simulink model "controls"  (R2022b)
settings: Solver=FixedStepAuto  StartTime=0.0  StopTime=inf  FixedStep=0.001  RelTol=1e-3
libraries: canmsglib x11, speedgoatlib_IO614 x5, speedgoatlib_CAN x1, battery_monitor_lib x1, driver_interface_lib x1, governor_lib x1, motor_interface_lib x1, simp_vd_lib x1
settings Model: Creator=maxfa  LastModifiedBy=maxfa
settings SolverCC: ConcurrentTasks=on  PositivePriorityOrder=on
settings OptimizationCC: BlockReduction=off  OptimizeBlockIOStorage=off
settings DebuggingCC: TasksWithSamePriorityMsg=none
settings HardwareCC: ProdBitPerLong=64  ProdLongLongMode=on  ProdHWDeviceType=Intel->x86-64 (Linux 64)
settings RTWCC: Description=Simulink Real-Time  SystemTargetFile=slrealtime.tlc  TemplateMakefile=slrealtime_default_tmf  Toolchain=Simulink Real-Time Toolchain  BuildConfiguration=Faster Runs  CodeExecutionProfiling=on  TargetLang=C++

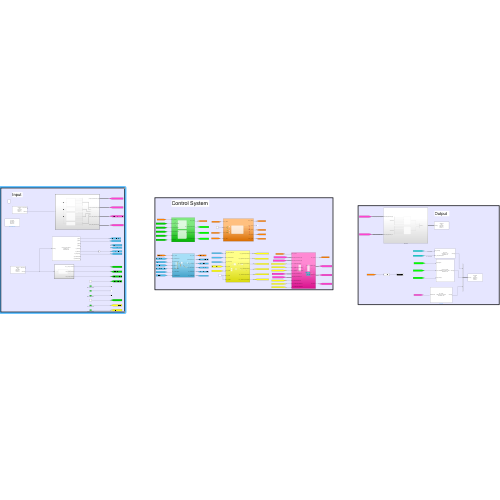
[thumbnail: Simulink's stored preview of the top-level diagram]
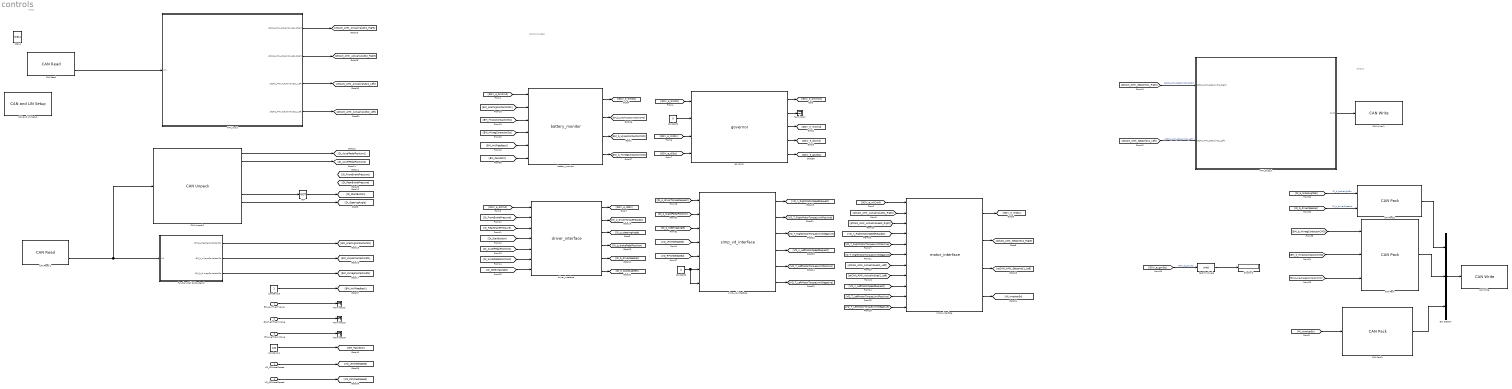
== system controls ==
  note: Control System
  note: Input
  note: Output
  BM_LowThermValue : Inport  OutDataTypeStr=int8  Unit=°C
  BM_HighThermValue : Inport  Port=2  OutDataTypeStr=int8  Unit=°C
  BM_AvgThermValue : Inport  Port=3  OutDataTypeStr=int8  Unit=°C
  VD_LFWheelSpeed : Inport  Port=4  OutDataTypeStr=int16  Unit=rpm
  VD_RFWheelSpeed : Inport  Port=5  OutDataTypeStr=int16  Unit=rpm
  AMK_Input : Subsystem  TreatAsAtomicUnit=on
  AMK_Output : Subsystem
  Bus Creator : BusCreator  Inputs=3
  CAN Pack : canmsglib/CAN Pack  CANdbFile=C:\Users\maxfa\Documents\MAC FE\can_dbc\dbcs\VEH_CAN.dbc  MsgList=Contactor_States  MsgName=Contactor_States  MsgIDType=Standard (11-bit identifier)  MsgIdentifier=1570  MsgLength=3  Remote=off  ApplyMinMax=off  BusOutput=off  SignalInfo={'Pack_Negative','16','8','LE','unsigned','Standard','0','1','0','-Inf','Inf';'Pack_Positive','0','8','LE','unsigned','Standard','0','1','0','-Inf','Inf';'Pack_Precharge','8','8','LE','unsigned','Standard','0','1','0','-Inf','Inf'}
      settings: LibrarySourceBlock=canlib/CAN Pack  DataFormat=CANdb specified signals
  CAN Pack1 : canmsglib/CAN Pack  CANdbFile=C:\Users\maxfa\Documents\MAC FE\racecar\firmware\dbcs\veh.dbc  MsgList=InverterCommand  MsgName=InverterCommand  MsgIDType=Standard (11-bit identifier)  MsgIdentifier=1560  MsgLength=1  Remote=off  ApplyMinMax=off  BusOutput=off  SignalInfo={ 'EnableInverter', '0', '1', 'LE', 'unsigned', 'Standard', '0', '1', '0', '-Inf', 'Inf' }
      settings: LibrarySourceBlock=canlib/CAN Pack  DataFormat=CANdb specified signals
  CAN Pack2 : canmsglib/CAN Pack  CANdbFile=C:\Users\maxfa\Documents\MAC FE\racecar\firmware\dbcs\veh.dbc  MsgList=FC_cmd  MsgName=FC_cmd  MsgIDType=Standard (11-bit identifier)  MsgIdentifier=256  MsgLength=1  Remote=off  ApplyMinMax=off  BusOutput=off  SignalInfo={ 'FC_brakeLight', '0', '1', 'LE', 'unsigned', 'Standard', '0', '1', '0', '0', '1'; 'FC_readyToDriveSpeaker', '1', '1', 'LE', 'unsigned', 'Standard', '0', '1', '0', '0', '1' }
      settings: LibrarySourceBlock=canlib/CAN Pack  DataFormat=CANdb specified signals
  "CAN Read " : speedgoatlib_IO614/CAN Read   moduleType=IO614  id=1  channel=1  canType=CAN (HS)  useBusOut=off  HasMulRead=Single Read from Buffer (FIFO)  MsgIDlist=[1 2]  isEFF=off  LabelInHex=on  enableInput=off  ts=-1  initValues=[614 1 -1 0 1 1 0 0 0 1 2 1 2]
      settings: SourceProductName=Simulink Real-Time: Speedgoat I/O Blockset
  CAN Read 1 : speedgoatlib_IO614/CAN Read   moduleType=IO614  id=1  channel=2  canType=CAN (HS)  useBusOut=off  HasMulRead=Single Read from Buffer (FIFO)  MsgIDlist=[1 2]  isEFF=off  LabelInHex=on  enableInput=off  ts=-1  initValues=[614 1 -1 1 1 1 0 0 0 1 2 1 2]
      settings: SourceProductName=Simulink Real-Time: Speedgoat I/O Blockset
  CAN Unpack2 : canmsglib/CAN Unpack  CANdbFile=C:\Users\maxfa\Downloads\VEH_TEST_CAN.dbc  MsgList=fc_tx  MsgName=fc_tx  MsgIDType=Standard (11-bit identifier)  MsgIdentifier=256  MsgLength=8  SignalInfo={'fc_apps1','0','8','LE','unsigned','Standard','0','0.005','0','0','1';'fc_apps2','8','8','LE','unsigned','Standard','0','0.005','0','0','1';'fc_bpps1','16','8','LE','unsigned','Standard','0','0.005','0','0','1';'fc_bpps2','24','8','LE','unsigned','Standard','0','0.005','0','0','1';'fc_hvilStatus','41','1','LE','signed','Standard','0','1','0','0','1';'fc_startButton','40','1','LE','signed','Standard','0','1','0','0','1';'fc_steeringAngle','32','8','LE','unsigned','Standard','0','0.005','0','0','1';'vd_LFWheelSpeed','48','12','LE','signed','Standard','0','1','0','-2048','2047';'vd_RFWheelSpeed','60','12','LE','signed','Standard','0','1','0','-2048','2047'}  IDPort=off  TimestampPort=off  ErrorPort=off  RemotePort=off  LengthPort=off  StatusPort=off  ApplyMinMax=off
      settings: LibrarySourceBlock=canlib/CAN Unpack  DataFormat=CANdb specified signals
  "CAN Write " : speedgoatlib_IO614/CAN Write   moduleType=IO614  id=1  channel=2  canType=CAN (HS)  useBusIn=off  numOfMsg=3  enableInput=off  enableStatusPort=off  initValues=[614 1 -1 1 1 1 0 3 0 0]  ts=-1
      settings: SourceProductName=Simulink Real-Time: Speedgoat I/O Blockset
  CAN Write 1 : speedgoatlib_IO614/CAN Write   moduleType=IO614  id=1  channel=1  canType=CAN (HS)  useBusIn=off  numOfMsg=2  enableInput=off  enableStatusPort=off  initValues=[614 1 -1 0 1 1 0 2 0 0]  ts=-1
      settings: SourceProductName=Simulink Real-Time: Speedgoat I/O Blockset
  "CAN and LIN Setup " : speedgoatlib_IO614/CAN and LIN Setup   moduleInitValues="[614    1    1   -1   -1]"  id=1  moduleType=IO614  pciSlot=-1  canChn1=CAN (HS)  canChn2=CAN (HS)  canChn3=Disabled  canChn4=Disabled  linChn1=Disabled  linChn2=Disabled  canInitStructArray=[]  canTermStructArray=[]  canChn1InitValues="[2   4   1  31   8   2   1   5   2]"  arbBdrChn1=500 kBaud  arbManBdrChn1=[4,1,31,8]  fdBdrChn1=5.0 MBaud  fdManBdrChn1=[2,1,5,2]  canChn2InitValues="[2   4   1  31   8   2   1   5   2]"  arbBdrChn2=500 kBaud  arbManBdrChn2=[4,1,31,8]  fdBdrChn2=5.0 MBaud  fdManBdrChn2=[2,1,5,2]  canChn3InitValues="[1   2   1  31   8   2   1   5   2]"  arbBdrChn3=1.0 MBaud  arbManBdrChn3=[2,1,31,8]  fdBdrChn3=5.0 MBaud  fdManBdrChn3=[2,1,5,2]  canChn4InitValues="[1   2   1  31   8   2   1   5   2]"  arbBdrChn4=1.0 MBaud  arbManBdrChn4=[2,1,31,8]  fdBdrChn4=5.0 MBaud  fdManBdrChn4=[2,1,5,2]  bdrLIN1=19200  linChn1InitValues="[1  19200]"  bdrLIN2=19200  linChn2InitValues="[1  19200]"
      settings: LibrarySourceBlock=speedgoatlib_CANLIN_OfA2/CAN and LIN Setup
  Cast To Single : DataTypeConversion  OutDataTypeStr=uint8  SaturateOnIntegerOverflow=off  RndMeth=Floor
  Constant1 : Constant  Value=0
  Constant13 : Constant  OutMin=0  OutMax=1
  Constant14 : Constant  Value=100  OutMin=0  OutMax=100
  Constant2 : Constant  Value=0
  Display2 : Display
  Function-Call Subsystem2 : Subsystem  TreatAsAtomicUnit=on
  IO614 : speedgoatlib_CAN/IO614  SystemSampleTime=-1  VariantActivationTime=update diagram  Latency=0  AutoFrameSizeCalculation=off
      settings: SourceProductName=Simulink Real-Time: Speedgoat I/O Blockset
  NOT : Logic  Operator=NOT  IconShape=distinctive  AllPortsSameDT=off  OutDataTypeStr=boolean
  Terminator{,1..3} (4 alike) : Terminator
  battery_monitor : battery_monitor_lib/battery_monitor  SystemSampleTime=-1  VariantActivationTime=update diagram  Latency=0  AutoFrameSizeCalculation=off
  driver_interface : driver_interface_lib/driver_interface  SystemSampleTime=-1  VariantActivationTime=update diagram  Latency=0  AutoFrameSizeCalculation=off
  governor : governor_lib/governor  SystemSampleTime=-1  VariantActivationTime=update diagram  Latency=0  AutoFrameSizeCalculation=off
  motor_interface : motor_interface_lib/motor_interface  SystemSampleTime=-1  VariantActivationTime=update diagram  Latency=0  AutoFrameSizeCalculation=off
  simp_vd_interface : simp_vd_lib/simp_vd_interface  SystemSampleTime=-1  VariantActivationTime=update diagram  Latency=0  AutoFrameSizeCalculation=off
  wires:
  driver_interface/5 -> [DI_b_driverSpeaker]
  simp_vd_interface/6 -> [VD_T_LeftMotorTorqueLimitNegative]
  simp_vd_interface/5 -> [VD_T_LeftMotorTorqueLimitPositive]
  AMK_Input/4(ptCAN_AMK_ActualValues2_Left) -> [ptCAN_AMK_ActualValues2_Left]
  AMK_Output/1(Out1) -> CAN Write 1/1
  AMK_Input/3(ptCAN_AMK_ActualValues1_Left) -> [ptCAN_AMK_ActualValues1_Left]
  [VD_T_LeftMotorTorqueLimitPositive] -> motor_interface/10
  [BM_PackSOC] -> battery_monitor/6
  driver_interface/4 -> [DI_p_brakePedalPosition]
  motor_interface/4 -> [MI_InverterEn]
  [VD_T_LeftMotorTorqueLimitNegative] -> motor_interface/11
  motor_interface/3 -> [ptCAN_AMK_Setpoints1_Left]
  NOT/1 -> [DI_StartButton]
  motor_interface/2 -> [ptCAN_AMK_Setpoints1_Right]
  [DI_FrontBrakePressure] -> driver_interface/2
  [ptCAN_AMK_Setpoints1_Left] -> AMK_Output/2(ptCAN_AMK_Setpoints1_Left)  "ptCAN_AMK_Setpoints1_Left"
  simp_vd_interface/3 -> [VD_T_RightMotorTorqueLimitNegative]
  "CAN Read "/2 -> AMK_Input/1(In1)
  governor/2 -> Terminator/1
  CAN Read 1/2 -> Function-Call Subsystem2/1(In1), CAN Unpack2/1
  [VD_n_LeftMotorSpeedRequest] -> motor_interface/9
  [ptCAN_AMK_Setpoints1_Right] -> AMK_Output/1(ptCAN_AMK_Setpoints1_Right)  "ptCAN_AMK_Setpoints1_Right"
  AMK_Input/2(ptCAN_AMK_ActualValues2_Right) -> [ptCAN_AMK_ActualValues2_Right]
  AMK_Input/1(ptCAN_AMK_ActualValues1_Right) -> [ptCAN_AMK_ActualValues1_Right]
  [VD_T_RightMotorTorqueLimitPositive] -> motor_interface/5
  [DI_b_brakeLightEn] -> CAN Pack2/1  "DI_b_brakeLightEn"
  simp_vd_interface/1 -> [VD_n_RightMotorSpeedRequest]
  [ptCAN_AMK_ActualValues2_Left] -> motor_interface/8
  Function-Call Subsystem2/2(BM_b_HVposContactorSts) -> [BM_HVposContactorSts]
  [DI_AccelPedalPosition1] -> driver_interface/5
  CAN Unpack2/1 -> [DI_AccelPedalPosition1]
  [BM_b_HVnegContactorCMD] -> CAN Pack/1
  battery_monitor/1 -> [GOV_e_bmSts]
  Constant2/1 -> simp_vd_interface/7, simp_vd_interface/6
  [GOV_e_bmSts] -> governor/1
  [GOV_e_diCmd] -> driver_interface/1
  VD_RFWheelSpeed/1 -> [VD_RFWheelSpeed]
  [GOV_e_diSts] -> governor/4
  [VD_RFWheelSpeed] -> simp_vd_interface/5
  Constant1/1 -> governor/2
  CAN Unpack2/6 -> NOT/1
  [BM_HVnegContactorSts] -> battery_monitor/4
  driver_interface/1 -> [GOV_e_diSts]
  [DI_StartButton] -> driver_interface/4
  [GOV_e_bmCmd] -> battery_monitor/1
  governor/1 -> [GOV_e_bmCmd]
  [VD_T_RightMotorTorqueLimitNegative] -> motor_interface/6
  Cast To Single/1 -> Display2/1
  governor/3 -> [GOV_e_miCmd]
  [DI_b_driverSpeaker] -> CAN Pack2/2  "DI_b_driverSpeaker"
  [DI_p_driverTorqueRequest] -> simp_vd_interface/1
  [GOV_e_miSts] -> governor/3
  simp_vd_interface/2 -> [VD_T_RightMotorTorqueLimitPositive]
  CAN Unpack2/2 -> [DI_AccelPedalPosition2]
  [BM_prechrgContactorSts] -> battery_monitor/2
  [DI_p_steeringAngle] -> simp_vd_interface/3
  BM_LowThermValue/1 -> Terminator1/1
  [DI_RearBrakePressure] -> driver_interface/3
  battery_monitor/3 -> [BM_b_HVposContactorCMD]
  [BM_HVposContactorSts] -> battery_monitor/3
  [BM_HvilFeedback] -> battery_monitor/5
  simp_vd_interface/4 -> [VD_n_LeftMotorSpeedRequest]
  VD_LFWheelSpeed/1 -> [VD_LFWheelSpeed]
  [MI_InverterEn] -> CAN Pack1/1
  [GOV_e_miCmd] -> motor_interface/1
  driver_interface/6 -> [DI_b_brakeLightEn]
  [ptCAN_AMK_ActualValues1_Right] -> motor_interface/2
  Function-Call Subsystem2/3(BM_b_HVnegContactorSts) -> [BM_HVnegContactorSts]
  [GOV_e_govSts] -> Cast To Single/1  "GOV_e_govSts"
  driver_interface/2 -> [DI_p_driverTorqueRequest]
  [BM_b_HVposContactorCMD] -> CAN Pack/2
  driver_interface/3 -> [DI_p_steeringAngle]
  [DI_SteeringAngle] -> driver_interface/7
  battery_monitor/2 -> [BM_b_prechargeContactorCMD]
  governor/4 -> [GOV_e_diCmd]
  [DI_AccelPedalPosition2] -> driver_interface/6
  [ptCAN_AMK_ActualValues1_Left] -> motor_interface/7
  BM_HighThermValue/1 -> Terminator2/1
  [VD_n_RightMotorSpeedRequest] -> motor_interface/4
  BM_AvgThermValue/1 -> Terminator3/1
  Constant14/1 -> [BM_PackSOC]
  battery_monitor/4 -> [BM_b_HVnegContactorCMD]
  Constant13/1 -> [BM_HvilFeedback]
  motor_interface/1 -> [GOV_e_miSts]
  CAN Unpack2/7 -> [DI_SteeringAngle]
  [DI_p_brakePedalPosition] -> simp_vd_interface/2
  [BM_b_prechargeContactorCMD] -> CAN Pack/3
  [ptCAN_AMK_ActualValues2_Right] -> motor_interface/3
  Function-Call Subsystem2/1(BM_b_prechrgContactorSts) -> [BM_prechrgContactorSts]
  governor/5 -> [GOV_e_govSts]
  [VD_LFWheelSpeed] -> simp_vd_interface/4
  CAN Pack/1 -> Bus Creator/2
  CAN Pack1/1 -> Bus Creator/3
  Bus Creator/1 -> "CAN Write "/1
  CAN Pack2/1 -> Bus Creator/1

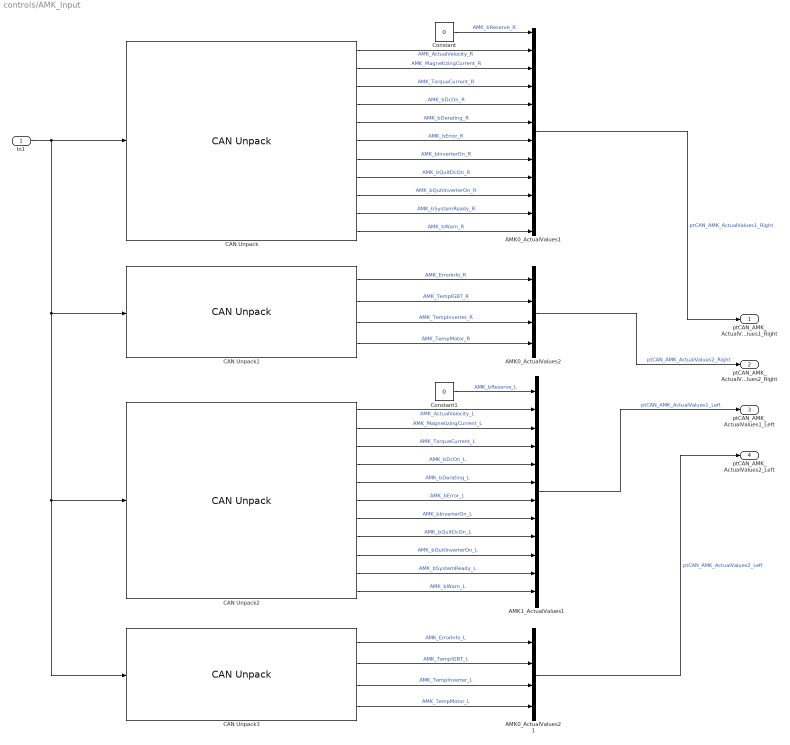
== system controls/AMK_Input ==
  In1 : Inport
  "AMK0_ActualValues1 " : BusCreator  Inputs=12
  "AMK0_ActualValues2 " : BusCreator  Inputs=4
  AMK0_ActualValues2 1 : BusCreator  Inputs=4
  AMK1_ActualValues1 : BusCreator  Inputs=12
  CAN Unpack : canmsglib/CAN Unpack  CANdbFile=C:\Users\maxfa\OneDrive\Documents\vehicle_control_system\src\testing\Plant\Bench\CAN_Databases-master\CAN_AMKInverter.dbc  MsgList=AMK1_ActualValues1  MsgName=AMK1_ActualValues1  MsgIDType=Standard (11-bit identifier)  MsgIdentifier=645  MsgLength=8  SignalInfo={'AMK_ActualVelocity','16','16','LE','signed','Standard','0','1','0','-Inf','Inf';'AMK_MagnetizingCurrent','48','16','LE','signed','Standard','0','1','0','-Inf','Inf';'AMK_TorqueCurrent','32','16','LE','signed','Standard','0','1','0','-Inf','Inf';'AMK_bDcOn','12','1','LE','unsigned','Standard','0','1','0','-Inf','Inf';'AMK_bDerating','15','1','LE','unsigned','Standard','0','1','0','-Inf','Inf';'AMK_bError','9','1','LE','unsigned','Standard','0','1','0','-Inf','Inf';'AMK_bInverterOn','14','1','LE','unsigned','Standard','0','1','0','-Inf','Inf';'AMK_bQuitDcOn','11','1','LE','unsigned','Standard','0','1','0','-Inf','Inf';'AMK_bQuitInverterOn','13','1','LE','unsigned','Standard','0','1','0','-Inf','Inf';'AMK_bSystemReady','8','1','LE','unsigned','Standard','0','1','0','-Inf','Inf';'AMK_bWarn','10','1','LE','unsigned','Standard','0','1','0','-Inf','Inf'}  IDPort=off  TimestampPort=off  ErrorPort=off  RemotePort=off  LengthPort=off  StatusPort=off  ApplyMinMax=off
      settings: LibrarySourceBlock=canlib/CAN Unpack  DataFormat=CANdb specified signals
  CAN Unpack1 : canmsglib/CAN Unpack  CANdbFile=C:\Users\maxfa\OneDrive\Documents\vehicle_control_system\src\testing\Plant\Bench\CAN_Databases-master\CAN_AMKInverter.dbc  MsgList=AMK1_ActualValues2  MsgName=AMK1_ActualValues2  MsgIDType=Standard (11-bit identifier)  MsgIdentifier=647  MsgLength=8  SignalInfo={'AMK_ErrorInfo','32','16','LE','unsigned','Standard','0','1','0','0','65535';'AMK_TempIGBT','48','16','LE','signed','Standard','0','0.1','0','-3276.8','3276.7';'AMK_TempInverter','16','16','LE','signed','Standard','0','0.1','0','-3276.8','3276.7';'AMK_TempMotor','0','16','LE','signed','Standard','0','0.1','0','-3276.8','3276.7'}  IDPort=off  TimestampPort=off  ErrorPort=off  RemotePort=off  LengthPort=off  StatusPort=off  ApplyMinMax=off
      settings: LibrarySourceBlock=canlib/CAN Unpack  DataFormat=CANdb specified signals
  CAN Unpack2 : canmsglib/CAN Unpack  CANdbFile=C:\Users\maxfa\OneDrive\Documents\vehicle_control_system\src\testing\Plant\Bench\CAN_Databases-master\CAN_AMKInverter.dbc  MsgList=AMK0_ActualValues1  MsgName=AMK0_ActualValues1  MsgIDType=Standard (11-bit identifier)  MsgIdentifier=644  MsgLength=8  SignalInfo={'AMK_ActualVelocity','16','16','LE','signed','Standard','0','1','0','-Inf','Inf';'AMK_MagnetizingCurrent','48','16','LE','signed','Standard','0','1','0','-Inf','Inf';'AMK_TorqueCurrent','32','16','LE','signed','Standard','0','1','0','-Inf','Inf';'AMK_bDcOn','12','1','LE','unsigned','Standard','0','1','0','-Inf','Inf';'AMK_bDerating','15','1','LE','unsigned','Standard','0','1','0','-Inf','Inf';'AMK_bError','9','1','LE','unsigned','Standard','0','1','0','-Inf','Inf';'AMK_bInverterOn','14','1','LE','unsigned','Standard','0','1','0','-Inf','Inf';'AMK_bQuitDcOn','11','1','LE','unsigned','Standard','0','1','0','-Inf','Inf';'AMK_bQuitInverterOn','13','1','LE','unsigned','Standard','0','1','0','-Inf','Inf';'AMK_bSystemReady','8','1','LE','unsigned','Standard','0','1','0','-Inf','Inf';'AMK_bWarn','10','1','LE','unsigned','Standard','0','1','0','-Inf','Inf'}  IDPort=off  TimestampPort=off  ErrorPort=off  RemotePort=off  LengthPort=off  StatusPort=off  ApplyMinMax=off
      settings: LibrarySourceBlock=canlib/CAN Unpack  DataFormat=CANdb specified signals
  CAN Unpack3 : canmsglib/CAN Unpack  CANdbFile=C:\Users\maxfa\OneDrive\Documents\vehicle_control_system\src\testing\Plant\Bench\CAN_Databases-master\CAN_AMKInverter.dbc  MsgList=AMK0_ActualValues2  MsgName=AMK0_ActualValues2  MsgIDType=Standard (11-bit identifier)  MsgIdentifier=646  MsgLength=8  SignalInfo={'AMK_ErrorInfo','32','16','LE','unsigned','Standard','0','1','0','0','65535';'AMK_TempIGBT','48','16','LE','signed','Standard','0','0.1','0','-3276.8','3276.7';'AMK_TempInverter','16','16','LE','signed','Standard','0','0.1','0','-3276.8','3276.7';'AMK_TempMotor','0','16','LE','signed','Standard','0','0.1','0','-3276.8','3276.7'}  IDPort=off  TimestampPort=off  ErrorPort=off  RemotePort=off  LengthPort=off  StatusPort=off  ApplyMinMax=off
      settings: LibrarySourceBlock=canlib/CAN Unpack  DataFormat=CANdb specified signals
  Constant : Constant  Value=0
  Constant1 : Constant  Value=0
  ptCAN_AMK_ActualValues1_Right : Outport
  ptCAN_AMK_ActualValues2_Right : Outport  Port=2
  ptCAN_AMK_ActualValues1_Left : Outport  Port=3
  ptCAN_AMK_ActualValues2_Left : Outport  Port=4
  wires:
  In1/1 -> CAN Unpack3/1, CAN Unpack2/1, CAN Unpack1/1, CAN Unpack/1
  CAN Unpack/1 -> "AMK0_ActualValues1 "/2  "AMK_ActualVelocity_R"
  CAN Unpack/2 -> "AMK0_ActualValues1 "/3  "AMK_MagnetizingCurrent_R"
  CAN Unpack/3 -> "AMK0_ActualValues1 "/4  "AMK_TorqueCurrent_R"
  CAN Unpack/4 -> "AMK0_ActualValues1 "/5  "AMK_bDcOn_R"
  CAN Unpack/5 -> "AMK0_ActualValues1 "/6  "AMK_bDerating_R"
  CAN Unpack/6 -> "AMK0_ActualValues1 "/7  "AMK_bError_R"
  CAN Unpack/7 -> "AMK0_ActualValues1 "/8  "AMK_bInverterOn_R"
  CAN Unpack/8 -> "AMK0_ActualValues1 "/9  "AMK_bQuitDcOn_R"
  CAN Unpack/9 -> "AMK0_ActualValues1 "/10  "AMK_bQuitInverterOn_R"
  CAN Unpack/10 -> "AMK0_ActualValues1 "/11  "AMK_bSystemReady_R"
  CAN Unpack/11 -> "AMK0_ActualValues1 "/12  "AMK_bWarn_R"
  "AMK0_ActualValues1 "/1 -> ptCAN_AMK_ActualValues1_Right/1  "ptCAN_AMK_ActualValues1_Right"
  CAN Unpack2/1 -> AMK1_ActualValues1/2  "AMK_ActualVelocity_L"
  CAN Unpack2/10 -> AMK1_ActualValues1/11  "AMK_bSystemReady_L"
  CAN Unpack2/6 -> AMK1_ActualValues1/7  "AMK_bError_L"
  CAN Unpack2/9 -> AMK1_ActualValues1/10  "AMK_bQuitInverterOn_L"
  CAN Unpack2/2 -> AMK1_ActualValues1/3  "AMK_MagnetizingCurrent_L"
  CAN Unpack2/3 -> AMK1_ActualValues1/4  "AMK_TorqueCurrent_L"
  AMK1_ActualValues1/1 -> ptCAN_AMK_ActualValues1_Left/1  "ptCAN_AMK_ActualValues1_Left"
  CAN Unpack2/8 -> AMK1_ActualValues1/9  "AMK_bQuitDcOn_L"
  CAN Unpack2/4 -> AMK1_ActualValues1/5  "AMK_bDcOn_L"
  CAN Unpack2/5 -> AMK1_ActualValues1/6  "AMK_bDerating_L"
  CAN Unpack2/11 -> AMK1_ActualValues1/12  "AMK_bWarn_L"
  CAN Unpack2/7 -> AMK1_ActualValues1/8  "AMK_bInverterOn_L"
  CAN Unpack1/1 -> "AMK0_ActualValues2 "/1  "AMK_ErrorInfo_R"
  CAN Unpack1/2 -> "AMK0_ActualValues2 "/2  "AMK_TempIGBT_R"
  CAN Unpack1/3 -> "AMK0_ActualValues2 "/3  "AMK_TempInverter_R"
  CAN Unpack1/4 -> "AMK0_ActualValues2 "/4  "AMK_TempMotor_R"
  "AMK0_ActualValues2 "/1 -> ptCAN_AMK_ActualValues2_Right/1  "ptCAN_AMK_ActualValues2_Right"
  CAN Unpack3/1 -> AMK0_ActualValues2 1/1  "AMK_ErrorInfo_L"
  CAN Unpack3/4 -> AMK0_ActualValues2 1/4  "AMK_TempMotor_L"
  AMK0_ActualValues2 1/1 -> ptCAN_AMK_ActualValues2_Left/1  "ptCAN_AMK_ActualValues2_Left"
  CAN Unpack3/3 -> AMK0_ActualValues2 1/3  "AMK_TempInverter_L"
  CAN Unpack3/2 -> AMK0_ActualValues2 1/2  "AMK_TempIGBT_L"
  Constant/1 -> "AMK0_ActualValues1 "/1  "AMK_bReserve_R"
  Constant1/1 -> AMK1_ActualValues1/1  "AMK_bReserve_L"

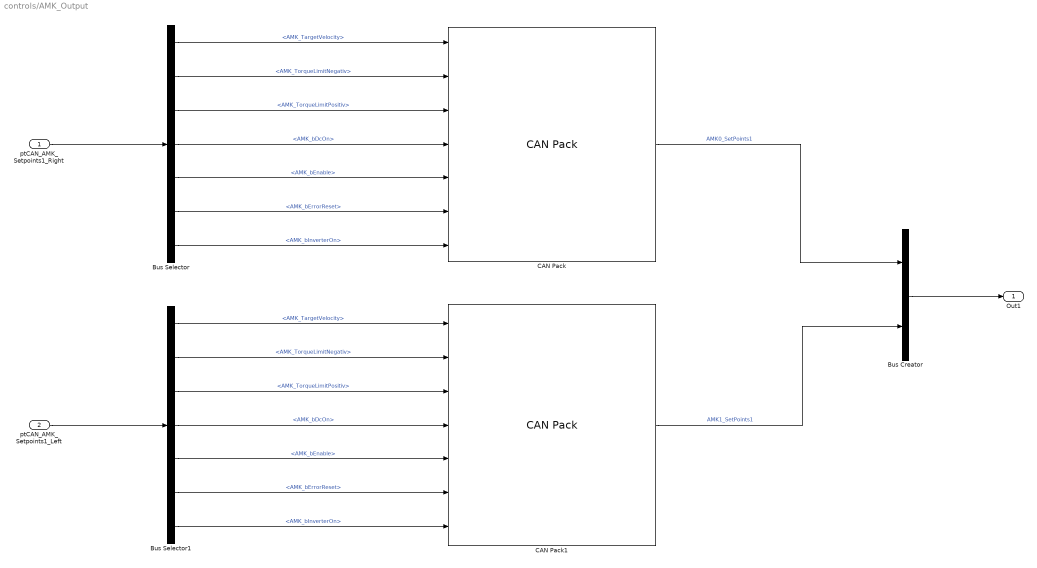
== system controls/AMK_Output ==
  ptCAN_AMK_Setpoints1_Right : Inport
  ptCAN_AMK_Setpoints1_Left : Inport  Port=2
  Bus Creator : BusCreator  Inputs=2
  Bus Selector : BusSelector  OutputSignals=AMK_TargetVelocity,AMK_TorqueLimitNegativ,AMK_TorqueLimitPositiv,AMK_bDcOn,AMK_bEnable,AMK_bErrorReset,AMK_bInverterOn
  Bus Selector1 : BusSelector  OutputSignals=AMK_TargetVelocity,AMK_TorqueLimitNegativ,AMK_TorqueLimitPositiv,AMK_bDcOn,AMK_bEnable,AMK_bErrorReset,AMK_bInverterOn
  CAN Pack : canmsglib/CAN Pack  CANdbFile=C:\Users\maxfa\OneDrive\Documents\vehicle_control_system\src\testing\Plant\Bench\CAN_Databases-master\CAN_AMKInverter.dbc  MsgList=AMK1_SetPoints1  MsgName=AMK1_SetPoints1  MsgIDType=Standard (11-bit identifier)  MsgIdentifier=390  MsgLength=8  Remote=off  ApplyMinMax=off  BusOutput=off  SignalInfo={'AMK_TargetVelocity','16','16','LE','signed','Standard','0','1','0','-Inf','Inf';'AMK_TorqueLimitNegativ','48','16','LE','signed','Standard','0','1','0','-Inf','Inf';'AMK_TorqueLimitPositiv','32','16','LE','signed','Standard','0','1','0','-Inf','Inf';'AMK_bDcOn','9','1','LE','unsigned','Standard','0','1','0','-Inf','Inf';'AMK_bEnable','10','1','LE','unsigned','Standard','0','1','0','-Inf','Inf';'AMK_bErrorReset','11','1','LE','unsigned','Standard','0','1','0','-Inf','Inf';'AMK_bInverterOn','8','1','LE','unsigned','Standard','0','1','0','-Inf','Inf'}
      settings: LibrarySourceBlock=canlib/CAN Pack  DataFormat=CANdb specified signals
  CAN Pack1 : canmsglib/CAN Pack  CANdbFile=C:\Users\maxfa\OneDrive\Documents\vehicle_control_system\src\testing\Plant\Bench\CAN_Databases-master\CAN_AMKInverter.dbc  MsgList=AMK0_SetPoints1  MsgName=AMK0_SetPoints1  MsgIDType=Standard (11-bit identifier)  MsgIdentifier=389  MsgLength=8  Remote=off  ApplyMinMax=off  BusOutput=off  SignalInfo={'AMK_TargetVelocity','16','16','LE','signed','Standard','0','1','0','-Inf','Inf';'AMK_TorqueLimitNegativ','48','16','LE','signed','Standard','0','1','0','-Inf','Inf';'AMK_TorqueLimitPositiv','32','16','LE','signed','Standard','0','1','0','-Inf','Inf';'AMK_bDcOn','9','1','LE','unsigned','Standard','0','1','0','-Inf','Inf';'AMK_bEnable','10','1','LE','unsigned','Standard','0','1','0','-Inf','Inf';'AMK_bErrorReset','11','1','LE','unsigned','Standard','0','1','0','-Inf','Inf';'AMK_bInverterOn','8','1','LE','unsigned','Standard','0','1','0','-Inf','Inf'}
      settings: LibrarySourceBlock=canlib/CAN Pack  DataFormat=CANdb specified signals
  Out1 : Outport
  wires:
  CAN Pack/1 -> Bus Creator/1  "AMK0_SetPoints1"
  CAN Pack1/1 -> Bus Creator/2  "AMK1_SetPoints1"
  Bus Selector/7 -> CAN Pack/7  "<AMK_bInverterOn>"
  Bus Selector/4 -> CAN Pack/4  "<AMK_bDcOn>"
  Bus Selector/5 -> CAN Pack/5  "<AMK_bEnable>"
  Bus Selector/6 -> CAN Pack/6  "<AMK_bErrorReset>"
  Bus Selector/1 -> CAN Pack/1  "<AMK_TargetVelocity>"
  Bus Selector/3 -> CAN Pack/3  "<AMK_TorqueLimitPositiv>"
  Bus Selector/2 -> CAN Pack/2  "<AMK_TorqueLimitNegativ>"
  Bus Creator/1 -> Out1/1
  Bus Selector1/1 -> CAN Pack1/1  "<AMK_TargetVelocity>"
  Bus Selector1/3 -> CAN Pack1/3  "<AMK_TorqueLimitPositiv>"
  Bus Selector1/2 -> CAN Pack1/2  "<AMK_TorqueLimitNegativ>"
  Bus Selector1/4 -> CAN Pack1/4  "<AMK_bDcOn>"
  Bus Selector1/5 -> CAN Pack1/5  "<AMK_bEnable>"
  Bus Selector1/6 -> CAN Pack1/6  "<AMK_bErrorReset>"
  Bus Selector1/7 -> CAN Pack1/7  "<AMK_bInverterOn>"
  ptCAN_AMK_Setpoints1_Right/1 -> Bus Selector/1
  ptCAN_AMK_Setpoints1_Left/1 -> Bus Selector1/1

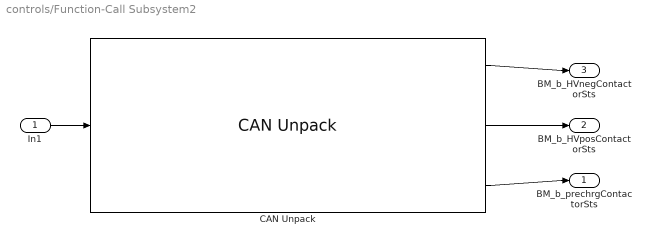
== system controls/Function-Call Subsystem2 ==
  In1 : Inport
  CAN Unpack : canmsglib/CAN Unpack  CANdbFile=C:\Users\maxfa\Documents\MAC FE\can_dbc\dbcs\VEH_CAN.dbc  MsgList=Contactor_Feedback  MsgName=Contactor_Feedback  MsgIDType=Standard (11-bit identifier)  MsgIdentifier=1574  MsgLength=3  SignalInfo={'Pack_Negative_Feedback','8','1','LE','unsigned','Standard','0','1','0','0','1';'Pack_Positive_Feedback','0','1','LE','unsigned','Standard','0','1','0','0','1';'Pack_Precharge_Feedback','16','1','LE','unsigned','Standard','0','1','0','0','1'}  IDPort=off  TimestampPort=off  ErrorPort=off  RemotePort=off  LengthPort=off  StatusPort=off  ApplyMinMax=off
      settings: LibrarySourceBlock=canlib/CAN Unpack  DataFormat=CANdb specified signals
  BM_b_prechrgContactorSts : Outport
  BM_b_HVposContactorSts : Outport  Port=2
  BM_b_HVnegContactorSts : Outport  Port=3
  wires:
  CAN Unpack/3 -> BM_b_prechrgContactorSts/1
  In1/1 -> CAN Unpack/1
  CAN Unpack/2 -> BM_b_HVposContactorSts/1
  CAN Unpack/1 -> BM_b_HVnegContactorSts/1
